simulink model "ControladorLateral"  (Simulink 8.2)
settings: Solver=ode3  StartTime=0.0  StopTime=3  FixedStep=0.005  RelTol=1e-3
InitFcn:
  | Alt = 2;
  | Vel =4;
  | wa = 72;
  | zetaA = 0.7;
  | load('../../Ganhos/BV9_30_03/GanhosTanqueHalf')
  | load('../../Dados_Input_Ganhos/BV9_30_03/sstanqueHalf_0')
  | [n,d] = butter(2,15*2*pi,'s')
  | F = tf(n,d);
  | Fd = c2d(F,0.01,'tustin');
  | [num, dem] = tfdata(Fd);
  | Ta = 100;
undefined symbols (not defined in the file or in its folder): Kd, Kp, Log, Plano_Lat
libraries: simulink x2
settings Model: Creator=AGSilva  LastModifiedBy=agsilva
settings OptimizationCC: InitFltsAndDblsToZero=on
settings DebuggingCC: SaveWithParameterizedLinksMsg=none
settings SFSimCC: SimParseCustomCode=off
settings GRTTargetCC: TargetFcnLib=ansi_tfl_tmw.mat

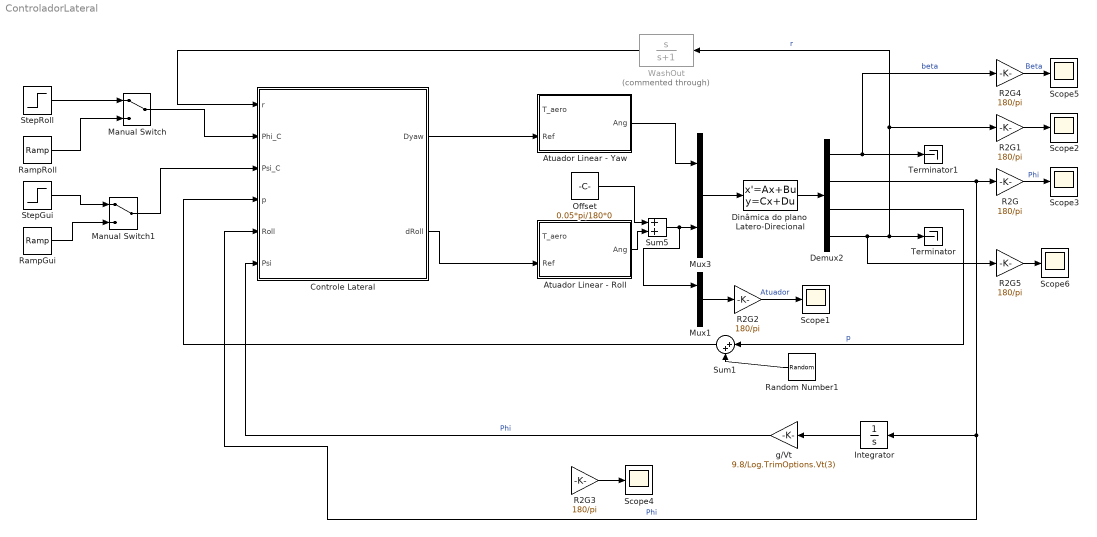
== system ControladorLateral ==
  Atuador Linear - Roll : Subsystem
  Atuador Linear - Yaw : Subsystem
  Controle Lateral : Subsystem
  Demux2 : Demux
  Dinâmica do plano  Latero-Direcional : StateSpace  A=Plano_Lat(Alt,Vel).A  B=Plano_Lat(Alt,Vel).B  C=eye(4)  D=zeros(4,2)  X0=[0 0 0 0*10*pi/180]
  Integrator : Integrator
  Manual Switch : ManualSwitch
  Manual Switch1 : ManualSwitch
  Mux1 : Mux  Inputs=2
  Mux3 : Mux  Inputs=2
  Offset : Constant  Value=0.05*pi/180*0
  R2G{,1..5} (6 alike) : Gain  Gain=180/pi
  RampGui : simulink/Sources/Ramp  slope=2*pi/180  start=0  X0=0
  RampRoll : simulink/Sources/Ramp  slope=10*pi/180  start=0  X0=0
  Random Number1 : RandomNumber  Variance=(0.002)^2*0  SampleTime=0.005
  Scope{1..6} (6 alike) : Scope
      Scope3 settings: SaveName=ScopeData3
      Scope4 settings: SaveName=ScopeData2
      Scope5 settings: SaveName=ScopeData4
      Scope6 settings: SaveName=ScopeData5
  StepGui : Step  Time=0  After=5*pi/180*0  SampleTime=0
  StepRoll : Step  Time=0  After=10*pi/180*1  SampleTime=0
  Sum1 : Sum  Inputs=|++
  Sum5 : Sum
  Terminator : Terminator
  Terminator1 : Terminator
  WashOut : TransferFcn  Commented=through  Numerator=[1 0]  Denominator=[1 1]
  g/Vt : Gain  Gain=9.8/Log.TrimOptions.Vt(3)
  wires:
  Dinâmica do plano  Latero-Direcional/1 -> Demux2/1
  Demux2/2 -> Controle Lateral/5(Roll), Integrator/1, R2G/1  "Phi"
  Random Number1/1 -> Sum1/2
  Demux2/3 -> Sum1/1  "p"
  Demux2/4 -> R2G5/1, WashOut/1, R2G1/1, Terminator/1  "r"
  Mux3/1 -> Dinâmica do plano  Latero-Direcional/1
  R2G/1 -> Scope3/1  "Phi"
  R2G1/1 -> Scope2/1
  Atuador Linear - Yaw/1(Ang) -> Mux3/1
  R2G2/1 -> Scope1/1  "Atuador"
  Mux1/1 -> R2G2/1
  Sum5/1 -> Mux1/1, Mux3/2
  Offset/1 -> Sum5/1
  Atuador Linear - Roll/1(Ang) -> Sum5/2
  Integrator/1 -> g/Vt/1
  R2G3/1 -> Scope4/1
  Demux2/1 -> R2G4/1, Terminator1/1  "beta"
  R2G4/1 -> Scope5/1  "Beta"
  R2G5/1 -> Scope6/1
  WashOut/1 -> Controle Lateral/1(r)
  Sum1/1 -> Controle Lateral/4(p)
  g/Vt/1 -> Controle Lateral/6(Psi)  "Phi"
  Controle Lateral/1(Dyaw) -> Atuador Linear - Yaw/2(Ref)
  Controle Lateral/2(dRoll) -> Atuador Linear - Roll/2(Ref)
  StepRoll/1 -> Manual Switch/1
  RampRoll/1 -> Manual Switch/2
  Manual Switch/1 -> Controle Lateral/2(Phi_C)
  StepGui/1 -> Manual Switch1/1
  Manual Switch1/1 -> Controle Lateral/3(Psi_C)
  RampGui/1 -> Manual Switch1/2

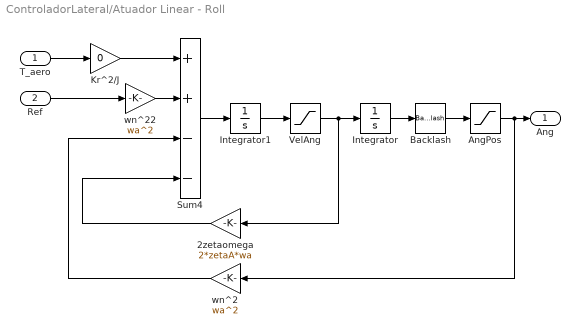
== system ControladorLateral/Atuador Linear - Roll ==
  T_aero : Inport
  Ref : Inport  Port=2
  2zetaomega : Gain  Gain=2*zetaA*wa
  AngPos : Saturate  UpperLimit=10*pi/180*10  LowerLimit=-10*pi/180*10
  Backlash : Backlash  BacklashWidth=0.05*pi/180*0
  Integrator : Integrator
  Integrator1 : Integrator
  Kr^2/J : Gain  Gain=0
  Sum4 : Sum  Inputs=++--
  VelAng : Saturate  UpperLimit=140*pi/180*10  LowerLimit=-140*pi/180*10
  wn^2 : Gain  Gain=wa^2
  wn^22 : Gain  Gain=wa^2
  Ang : Outport
  wires:
  2zetaomega/1 -> Sum4/4
  T_aero/1 -> Kr^2/J/1
  Ref/1 -> wn^22/1
  wn^2/1 -> Sum4/3
  Sum4/1 -> Integrator1/1
  Integrator/1 -> Backlash/1
  AngPos/1 -> wn^2/1, Ang/1
  Integrator1/1 -> VelAng/1
  wn^22/1 -> Sum4/2
  VelAng/1 -> 2zetaomega/1, Integrator/1
  Kr^2/J/1 -> Sum4/1
  Backlash/1 -> AngPos/1

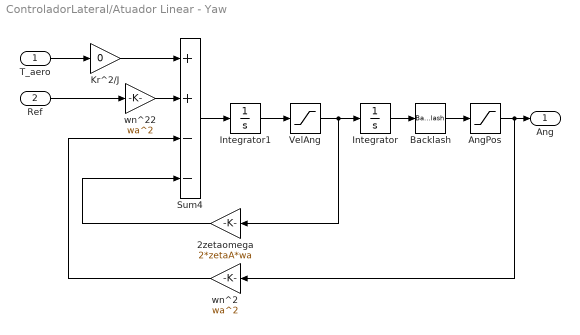
== system ControladorLateral/Atuador Linear - Yaw ==
  T_aero : Inport
  Ref : Inport  Port=2
  2zetaomega : Gain  Gain=2*zetaA*wa
  AngPos : Saturate  UpperLimit=10*pi/180  LowerLimit=-10*pi/180
  Backlash : Backlash  BacklashWidth=0.05*pi/180*0
  Integrator : Integrator
  Integrator1 : Integrator
  Kr^2/J : Gain  Gain=0
  Sum4 : Sum  Inputs=++--
  VelAng : Saturate  UpperLimit=140*pi/180  LowerLimit=-140*pi/180
  wn^2 : Gain  Gain=wa^2
  wn^22 : Gain  Gain=wa^2
  Ang : Outport
  wires:
  2zetaomega/1 -> Sum4/4
  T_aero/1 -> Kr^2/J/1
  Ref/1 -> wn^22/1
  wn^2/1 -> Sum4/3
  Sum4/1 -> Integrator1/1
  Integrator/1 -> Backlash/1
  AngPos/1 -> wn^2/1, Ang/1
  Integrator1/1 -> VelAng/1
  wn^22/1 -> Sum4/2
  VelAng/1 -> 2zetaomega/1, Integrator/1
  Kr^2/J/1 -> Sum4/1
  Backlash/1 -> AngPos/1

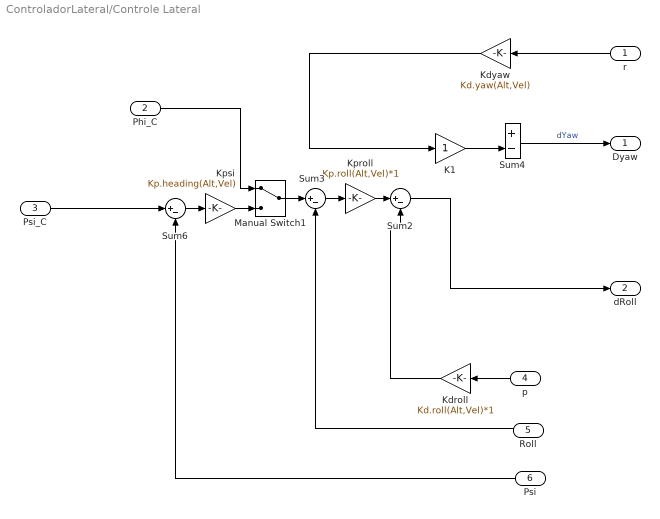
== system ControladorLateral/Controle Lateral ==
  r : Inport
  Phi_C : Inport  Port=2
  Psi_C : Inport  Port=3
  p : Inport  Port=4
  Roll : Inport  Port=5
  Psi : Inport  Port=6
  K1 : Gain
  "Kdroll " : Gain  Gain=Kd.roll(Alt,Vel)*1
  "Kdyaw " : Gain  Gain=Kd.yaw(Alt,Vel)
  Kproll : Gain  Gain=Kp.roll(Alt,Vel)*1
  Kpsi : Gain  Gain=Kp.heading(Alt,Vel)
  Manual Switch1 : ManualSwitch
  Sum2 : Sum  Inputs=|+-
  Sum3 : Sum  Inputs=|+-
  Sum4 : Sum  Inputs=+-
  Sum6 : Sum  Inputs=|+-
  Dyaw : Outport
  dRoll : Outport  Port=2
  wires:
  Sum3/1 -> Kproll/1
  Sum6/1 -> Kpsi/1
  Sum4/1 -> Dyaw/1  "dYaw"
  r/1 -> "Kdyaw "/1
  p/1 -> "Kdroll "/1
  Phi_C/1 -> Manual Switch1/1
  "Kdroll "/1 -> Sum2/2
  Kproll/1 -> Sum2/1
  Psi/1 -> Sum6/2
  Kpsi/1 -> Manual Switch1/2
  Manual Switch1/1 -> Sum3/1
  K1/1 -> Sum4/2
  Psi_C/1 -> Sum6/1
  Sum2/1 -> dRoll/1
  "Kdyaw "/1 -> K1/1
  Roll/1 -> Sum3/2
